simulink library "tanFrameProjection_ul"  (R2018b)
settings: Solver=VariableStepAuto  StartTime=0.0  StopTime=10.0  RelTol=1e-3
libraries: gnd2TanRotation_ul x1
settings Model: Creator=mcobb  LastModifiedBy=mcobb

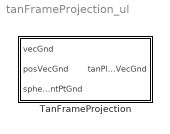
== system tanFrameProjection_ul ==
  TanFrameProjection : Subsystem

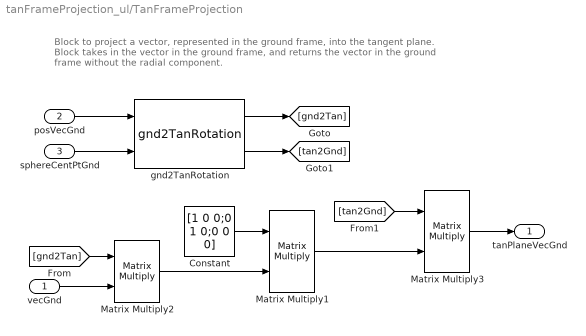
== system tanFrameProjection_ul/TanFrameProjection ==
  note: Block to project a vector, represented in the ground frame, into the tangent plane.
      | Block takes in the vector in the ground frame, and returns the vector in the
      | ground frame without the radial component.
  vecGnd : Inport
  posVecGnd : Inport  Port=2
  sphereCentPtGnd : Inport  Port=3
  Constant : Constant  Value=[1 0 0;0 1 0;0 0 0]
  Matrix Multiply1 : Product  Multiplication=Matrix(*)
  Matrix Multiply2 : Product  Multiplication=Matrix(*)
  Matrix Multiply3 : Product  Multiplication=Matrix(*)
  gnd2TanRotation : gnd2TanRotation_ul/gnd2TanRotation  SystemSampleTime=-1
  tanPlaneVecGnd : Outport
  wires:
  Matrix Multiply2/1 -> Matrix Multiply1/2
  vecGnd/1 -> Matrix Multiply2/2
  Matrix Multiply3/1 -> tanPlaneVecGnd/1
  gnd2TanRotation/2 -> [tan2Gnd]
  posVecGnd/1 -> gnd2TanRotation/1
  sphereCentPtGnd/1 -> gnd2TanRotation/2
  gnd2TanRotation/1 -> [gnd2Tan]
  [gnd2Tan] -> Matrix Multiply2/1
  Constant/1 -> Matrix Multiply1/1
  Matrix Multiply1/1 -> Matrix Multiply3/2
  [tan2Gnd] -> Matrix Multiply3/1
